simulink model "prelookupTest"  (R2017a)
settings: Solver=VariableStepAuto  StartTime=0.0  StopTime=10.0  RelTol=1e-3
InitFcn:
  | initalize_test
values from neighbouring files (symbols this model uses):
  alpha = 15    [initalize_test.m]    (also in state_plot.m = VinfHistory.Data(1:end-1,2))
  delta_f = 40    [initalize_test.m]
  deltaCJ = 1    [initalize_test.m]
settings Model: Creator=Devansh  LastModifiedBy=Devansh

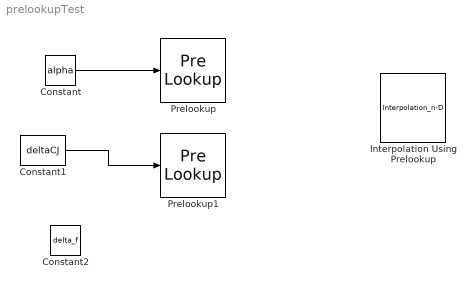
== system prelookupTest ==
  Constant : Constant  Value=alpha
  Constant1 : Constant  Value=deltaCJ
  Constant2 : Constant  Value=delta_f
  Interpolation Using Prelookup : Interpolation_n-D  InternalRulePriority=Speed
  Prelookup : PreLookup  BreakpointsData=alpha_vals  ExtrapMethod=Linear  DiagnosticForOutOfRangeInput=Warning
  Prelookup1 : PreLookup  BreakpointsData=deltaCJ_vals  ExtrapMethod=Linear  DiagnosticForOutOfRangeInput=Warning
  wires:
  Constant/1 -> Prelookup/1
  Constant1/1 -> Prelookup1/1
